simulink model "bank_angle_w_damping"  (R2017a)
settings: Solver=ode4  StartTime=0.0  StopTime=SimTime  FixedStep=stepSize  RelTol=1e-3
values from neighbouring files (symbols this model uses):
  tau = 0.125    [AE168_project.m]
undefined symbols (not defined in the file or in its folder): K_phi, K_phidot, phi_disturb, r_den, r_num
libraries: simulink_extras x3, dspsrcs4 x1
settings Model: Creator=Jeremiah  LastModifiedBy=Jeremiah

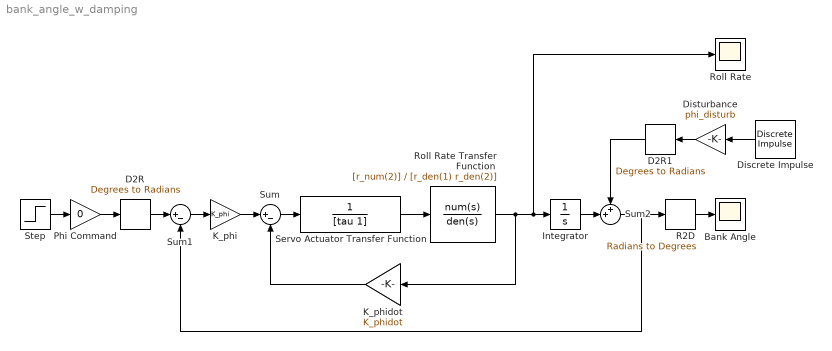
== system bank_angle_w_damping ==
  Bank Angle : Scope
  D2R : simulink_extras/Transformations/Degrees to Radians
  D2R1 : simulink_extras/Transformations/Degrees to Radians
  Discrete Impulse : dspsrcs4/Discrete  Impulse  Delay=0  SampleTime=0.5  FrameSample=1  OutputFrames=off  dataType=double  isSigned=on  wordLen=16  udDataType=sfix(16)  fracBitsMode=Best precision  numFracBits=15  OutDataTypeStr=double  LastOutDataTypeStr=double
  Disturbance : Gain  Gain=phi_disturb
  Integrator : Integrator
  K_phi : Gain  Gain=K_phi
  K_phidot : Gain  Gain=K_phidot
  Phi Command : Gain  Gain=0
  R2D : simulink_extras/Transformations/Radians to Degrees
  Roll Rate : Scope
  Roll Rate Transfer Function : TransferFcn  Numerator=[r_num(2)]  Denominator=[r_den(1) r_den(2)]  ContinuousStateAttributes='roll_rate'
  Servo Actuator Transfer Function : TransferFcn  Denominator=[tau 1]  ContinuousStateAttributes='pitch_attitude'
  Step : Step  Time=0  SampleTime=0.5
  Sum : Sum  Inputs=|+-
  Sum1 : Sum  Inputs=|+-
  Sum2 : Sum  Inputs=++|
  wires:
  Step/1 -> Phi Command/1
  Roll Rate Transfer Function/1 -> Integrator/1, Roll Rate/1, K_phidot/1
  R2D/1 -> Bank Angle/1
  Phi Command/1 -> D2R/1
  K_phidot/1 -> Sum/2
  Sum/1 -> Servo Actuator Transfer Function/1
  Sum1/1 -> K_phi/1
  K_phi/1 -> Sum/1
  D2R/1 -> Sum1/1
  Servo Actuator Transfer Function/1 -> Roll Rate Transfer Function/1
  Integrator/1 -> Sum2/2
  Sum2/1 -> Sum1/2, R2D/1
  D2R1/1 -> Sum2/1
  Disturbance/1 -> D2R1/1
  Discrete Impulse/1 -> Disturbance/1
